simulink model "21_MCU_dataLogger_simulation"  (R2023b)
settings: Solver=FixedStepDiscrete  StartTime=0.0  StopTime=10  FixedStep=50e-6  RelTol=1e-3
InitFcn:
  | % Sampling freq
  | Te = 0.5e-4 ;
  | 
  | % Electrical param
  | Rs = 0.6560; Ls = 3.5e-04;Ld = Ls; Lq = Ls; Phif= 0.0066;P= 4; Vemax=24;
  | 
  | % Mechanical param
  | J = 1e-5; f = 1e-5; Wrnom=2700*2*pi/60;
  | 
  | % State-space rep
  | A1c = [-Rs/(Ls) 0 ; 0 -Rs/(Ls)]; B1c= [1/(Ls) 0 ; 0 1/(Ls)]; C1c = [1 0 ; 0 1];
  | 
  | %Discretization
  | sys1d=c2d(ss(A1c, B1c, C1c, [0 0 ; 0 0]), Te, 'zoh');
  | [A1, B1, C1, D1]=ssdata(sys1d);
  | 
  | %DSMO param
  | h1 = 2/3; h2 = 15;
  | H1 = B1\A1*B1 + h1*eye(2); H2 = h2*eye(2); J_dsmo = [0 -1 ;  1 0];
  | 
  | % Adaptive obs param
  | gamma = 0.5/Te; h3 = 0.01; Telec = 2*pi/(Wrnom*P);fc = 3/(Telec);
undefined symbols (not defined in the file or in its folder): A1, B1
libraries: embmathops x1, simulink x1
Description:
  | Offline real-time high frequency data logging based methodology
  | for PMSM observer design
  | 
  | Alhak Hassan et al.
  | ELECTRIMACS 2024 – Castello de la Plana, Spain, 27-30 May 2024
settings Model: Creator=rdelpoux  LastModifiedBy=rdelpoux

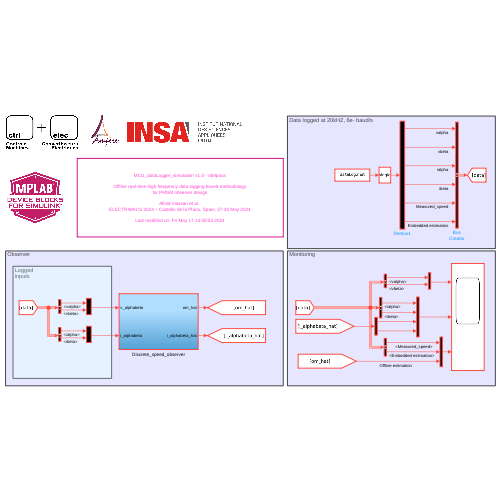
[thumbnail: Simulink's stored preview of the top-level diagram]
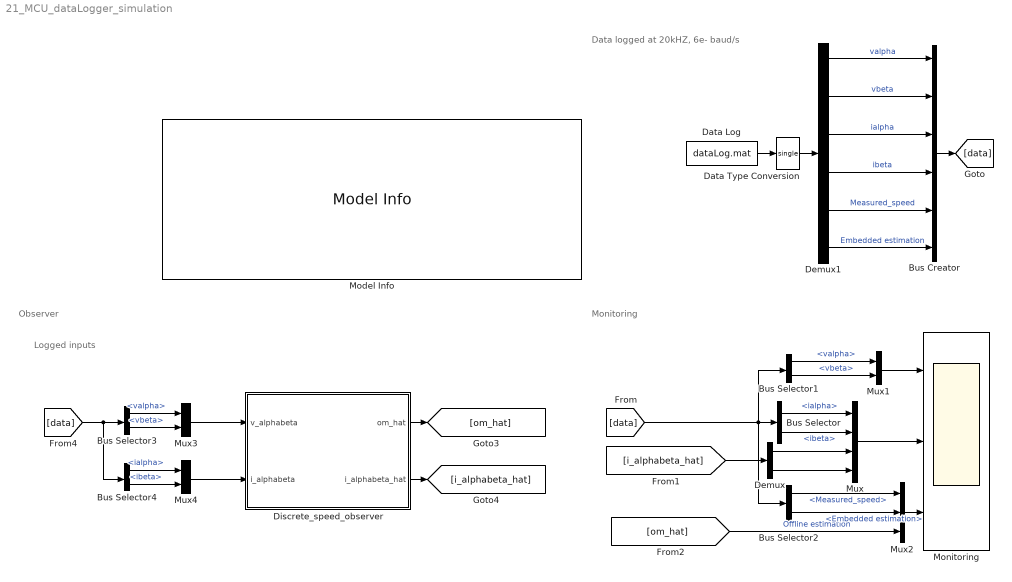
== system 21_MCU_dataLogger_simulation ==
  note: Logged
      | inputs
  note: Data logged at 20kHZ, 6e- baud/s
  note: Monitoring
  note: Observer
  Bus Creator : BusCreator  Inputs=6
  Bus Selector : BusSelector  OutputSignals=ialpha,ibeta
  Bus Selector1 : BusSelector  OutputSignals=valpha,vbeta
  Bus Selector2 : BusSelector  OutputSignals=Measured_speed,Embedded estimation
  Bus Selector3 : BusSelector  OutputSignals=valpha,vbeta
  Bus Selector4 : BusSelector  OutputSignals=ialpha,ibeta
  Data Log : FromFile  FileName=dataLog.mat  SampleTime=50e-6
  Data Type Conversion : DataTypeConversion  OutDataTypeStr=single  SaturateOnIntegerOverflow=off  RndMeth=Floor
  Demux : Demux  Outputs=2
  Demux1 : Demux  Outputs=6
  Discrete_speed_observer : Subsystem
  Model Info : simulink/Model-Wide Utilities/Model Info  Frame=on  DisplayStringWithTags=|  HorizontalTextAlignment=Center  LeftAlignmentValue=0.5
      | %<ModelName> v%<ModelVersion> - %<Creator>
      | 
      | %<Description>
      | 
      | Last modified on: %<LastModificationDate>
  Monitoring : Scope  NumInputPorts=3
  Mux : Mux
  Mux1 : Mux  Inputs=2
  Mux2 : Mux  Inputs=3
  Mux3 : Mux  Inputs=2
  Mux4 : Mux  Inputs=2
  wires:
  Data Log/1 -> Data Type Conversion/1
  Bus Creator/1 -> [data]
  Bus Selector/1 -> Mux/1  "<ialpha>"
  Bus Selector/2 -> Mux/2  "<ibeta>"
  Mux1/1 -> Monitoring/1
  Bus Selector1/2 -> Mux1/2  "<vbeta>"
  Bus Selector1/1 -> Mux1/1  "<valpha>"
  [data] -> Bus Selector/1, Bus Selector1/1, Bus Selector2/1
  Demux1/5 -> Bus Creator/5  "Measured_speed"
  Discrete_speed_observer/1(om_hat) -> [om_hat]
  [om_hat] -> Mux2/3  "Offline estimation"
  Data Type Conversion/1 -> Demux1/1
  Demux1/3 -> Bus Creator/3  "ialpha"
  Demux1/4 -> Bus Creator/4  "ibeta"
  Demux1/2 -> Bus Creator/2  "vbeta"
  Demux1/1 -> Bus Creator/1  "valpha"
  Demux1/6 -> Bus Creator/6  "Embedded estimation"
  Mux/1 -> Monitoring/2
  Bus Selector2/1 -> Mux2/1  "<Measured_speed>"
  Bus Selector2/2 -> Mux2/2  "<Embedded estimation>"
  Mux2/1 -> Monitoring/3
  Bus Selector3/1 -> Mux3/1  "<valpha>"
  Bus Selector3/2 -> Mux3/2  "<vbeta>"
  Mux3/1 -> Discrete_speed_observer/1(v_alphabeta)
  [data] -> Bus Selector4/1, Bus Selector3/1
  Bus Selector4/2 -> Mux4/2  "<ibeta>"
  Bus Selector4/1 -> Mux4/1  "<ialpha>"
  Mux4/1 -> Discrete_speed_observer/2(i_alphabeta)
  Discrete_speed_observer/2(i_alphabeta_hat) -> [i_alphabeta_hat]
  [i_alphabeta_hat] -> Demux/1
  Demux/1 -> Mux/3
  Demux/2 -> Mux/4

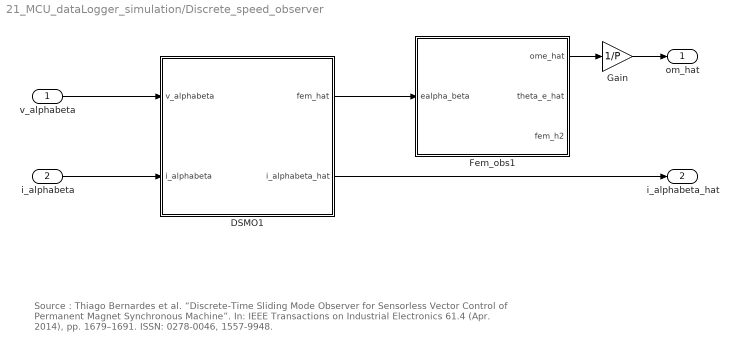
== system 21_MCU_dataLogger_simulation/Discrete_speed_observer ==
  note: Source : Thiago Bernardes et al. “Discrete-Time Sliding Mode Observer for Sensorless Vector Control of Permanent Magnet Synchronous Machine”. In: IEEE Transactions on Industrial Electronics 61.4 (Apr. 2014), pp. 1679–1691. ISSN: 0278-0046, 1557-9948.
  v_alphabeta : Inport
  i_alphabeta : Inport  Port=2
  DSMO1 : Subsystem
  Fem_obs1 : Subsystem
  Gain : Gain  Gain=1/P
  om_hat : Outport
  i_alphabeta_hat : Outport  Port=2
  wires:
  Fem_obs1/1(ome_hat) -> Gain/1
  i_alphabeta/1 -> DSMO1/2(i_alphabeta)
  v_alphabeta/1 -> DSMO1/1(v_alphabeta)
  DSMO1/1(fem_hat) -> Fem_obs1/1(ealpha_beta)
  Gain/1 -> om_hat/1
  DSMO1/2(i_alphabeta_hat) -> i_alphabeta_hat/1

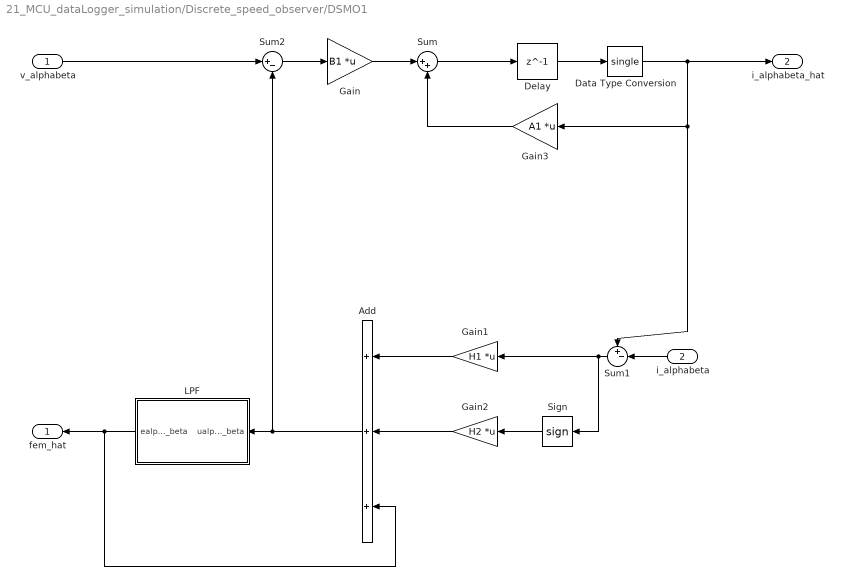
== system 21_MCU_dataLogger_simulation/Discrete_speed_observer/DSMO1 ==
  v_alphabeta : Inport
  i_alphabeta : Inport  Port=2
  Add : Sum  Inputs=+++
  Data Type Conversion : DataTypeConversion  OutDataTypeStr=single  SaturateOnIntegerOverflow=off  RndMeth=Floor
  Delay : Delay  DelayLength=1  InitialCondition=0  SampleTime=Te
  Gain : Gain  Gain=B1  Multiplication=Matrix(K*u)
  Gain1 : Gain  Gain=H1  Multiplication=Matrix(K*u)
  Gain2 : Gain  Gain=H2  Multiplication=Matrix(K*u)
  Gain3 : Gain  Gain=A1  Multiplication=Matrix(K*u)
  LPF : Subsystem
  Sign : Signum
  Sum : Sum  Inputs=|++
  Sum1 : Sum  Inputs=+-|
  Sum2 : Sum  Inputs=|+-
  fem_hat : Outport
  i_alphabeta_hat : Outport  Port=2
  wires:
  Data Type Conversion/1 -> Gain3/1, Sum1/1, i_alphabeta_hat/1
  Delay/1 -> Data Type Conversion/1
  Add/1 -> Sum2/2, LPF/1(ualpha_beta)
  LPF/1(ealpha_beta) -> fem_hat/1, Add/3
  Gain2/1 -> Add/2
  Sign/1 -> Gain2/1
  Gain1/1 -> Add/1
  Sum1/1 -> Gain1/1, Sign/1
  v_alphabeta/1 -> Sum2/1
  Sum2/1 -> Gain/1
  i_alphabeta/1 -> Sum1/2
  Gain3/1 -> Sum/2
  Gain/1 -> Sum/1
  Sum/1 -> Delay/1

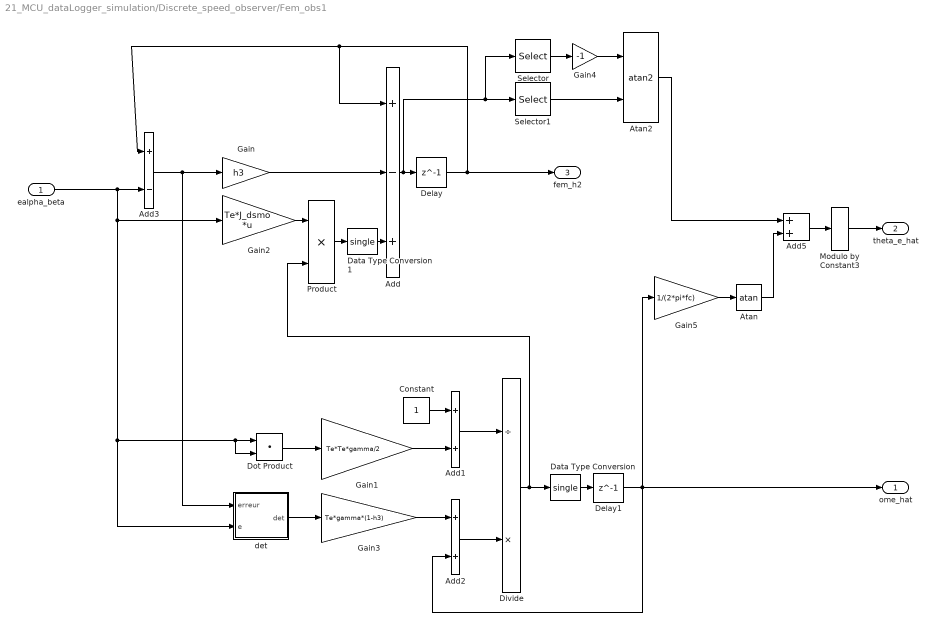
== system 21_MCU_dataLogger_simulation/Discrete_speed_observer/Fem_obs1 ==
  ealpha_beta : Inport
  Add : Sum  Inputs=+-+
  Add1 : Sum
  Add2 : Sum
  Add3 : Sum  Inputs=+-
  Add5 : Sum
  Atan : Trigonometry  Operator=atan
  Atan2 : Trigonometry  Operator=atan2  ApproximationMethod=Lookup  NumberOfDataPoints=32
  Constant : Constant
  Data Type Conversion : DataTypeConversion  OutDataTypeStr=single  SaturateOnIntegerOverflow=off  RndMeth=Floor
  Data Type Conversion1 : DataTypeConversion  OutDataTypeStr=single  SaturateOnIntegerOverflow=off  RndMeth=Floor
  Delay : Delay  DelayLength=1  SampleTime=Te
  Delay1 : Delay  DelayLength=1  SampleTime=Te
  Divide : Product  Inputs=/*
  Dot Product : DotProduct  OutDataTypeStr=Inherit: Inherit via internal rule
  Gain : Gain  Gain=h3
  Gain1 : Gain  Gain=Te*Te*gamma/2
  Gain2 : Gain  Gain=Te*J_dsmo  Multiplication=Matrix(K*u)
  Gain3 : Gain  Gain=Te*gamma*(1-h3)
  Gain4 : Gain  Gain=-1
  Gain5 : Gain  Gain=1/(2*pi*fc)
  Modulo by Constant3 : embmathops/Modulo by Constant  Denominator=2*pi  SimulateUsing=Code generation
      settings: LibrarySourceBlock=embeddedMathLib/Modulo by Constant
  Product : Product
  Selector : Selector  InputPortWidth=2  IndexOptions=Index vector (dialog)  Indices=[1]  OutputSizes=1
  Selector1 : Selector  InputPortWidth=2  IndexOptions=Index vector (dialog)  Indices=2  OutputSizes=1
  det : Subsystem
  ome_hat : Outport
  theta_e_hat : Outport  Port=2
  fem_h2 : Outport  Port=3
  wires:
  Modulo by Constant3/1 -> theta_e_hat/1
  Data Type Conversion1/1 -> Add/3
  Product/1 -> Data Type Conversion1/1
  Divide/1 -> Data Type Conversion/1, Product/2
  Data Type Conversion/1 -> Delay1/1
  Delay1/1 -> ome_hat/1, Add2/2, Gain5/1
  Add5/1 -> Modulo by Constant3/1
  Gain5/1 -> Atan/1
  Constant/1 -> Add1/1
  Atan/1 -> Add5/2
  Atan2/1 -> Add5/1
  Selector1/1 -> Atan2/2
  Gain4/1 -> Atan2/1
  Selector/1 -> Gain4/1
  Gain/1 -> Add/2
  ealpha_beta/1 -> Add3/2, Gain2/1, det/2(e), Dot Product/1, Dot Product/2
  Gain3/1 -> Add2/1
  det/1(det) -> Gain3/1
  Add2/1 -> Divide/2
  Gain1/1 -> Add1/2
  Add1/1 -> Divide/1
  Dot Product/1 -> Gain1/1
  Delay/1 -> fem_h2/1, Add3/1, Add/1
  Add/1 -> Selector/1, Selector1/1, Delay/1
  Gain2/1 -> Product/1
  Add3/1 -> det/1(erreur), Gain/1

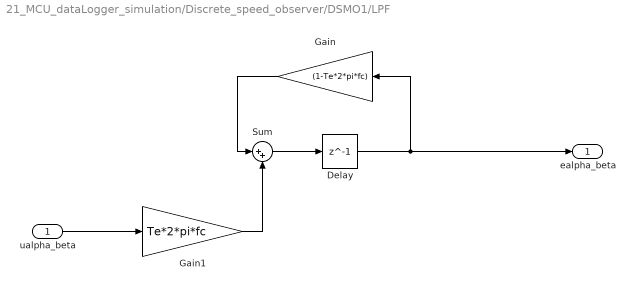
== system 21_MCU_dataLogger_simulation/Discrete_speed_observer/DSMO1/LPF ==
  ualpha_beta : Inport
  Delay : Delay  DelayLength=1  SampleTime=Te
  Gain : Gain  Gain=(1-Te*2*pi*fc)
  Gain1 : Gain  Gain=Te*2*pi*fc
  Sum : Sum  Inputs=|++
  ealpha_beta : Outport
  wires:
  ualpha_beta/1 -> Gain1/1
  Gain1/1 -> Sum/2
  Gain/1 -> Sum/1
  Delay/1 -> ealpha_beta/1, Gain/1
  Sum/1 -> Delay/1

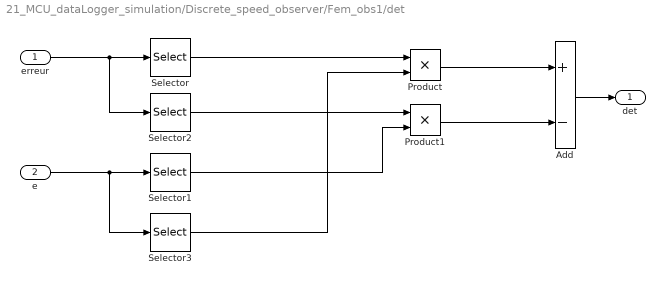
== system 21_MCU_dataLogger_simulation/Discrete_speed_observer/Fem_obs1/det ==
  erreur : Inport
  e : Inport  Port=2
  Add : Sum  Inputs=+-
  Product : Product
  Product1 : Product
  Selector : Selector  InputPortWidth=2  IndexOptions=Index vector (dialog)  Indices=[1]  OutputSizes=1
  Selector1 : Selector  InputPortWidth=2  IndexOptions=Index vector (dialog)  Indices=[1]  OutputSizes=1
  Selector2 : Selector  InputPortWidth=2  IndexOptions=Index vector (dialog)  Indices=[2]  OutputSizes=1
  Selector3 : Selector  InputPortWidth=2  IndexOptions=Index vector (dialog)  Indices=[2]  OutputSizes=1
  det : Outport
  wires:
  Add/1 -> det/1
  Product1/1 -> Add/2
  Selector1/1 -> Product1/2
  Selector2/1 -> Product1/1
  Product/1 -> Add/1
  Selector3/1 -> Product/2
  Selector/1 -> Product/1
  e/1 -> Selector1/1, Selector3/1
  erreur/1 -> Selector/1, Selector2/1
